simulink model "etb_Model"  (R2019b)
settings: Solver=FixedStepAuto  StartTime=0.0  StopTime=6  FixedStep=.001  RelTol=1e-3
undefined symbols (not defined in the file or in its folder): DiscIntNeverNeededParam
libraries: simulink x1
settings Model: Creator=Nick  LastModifiedBy=starw

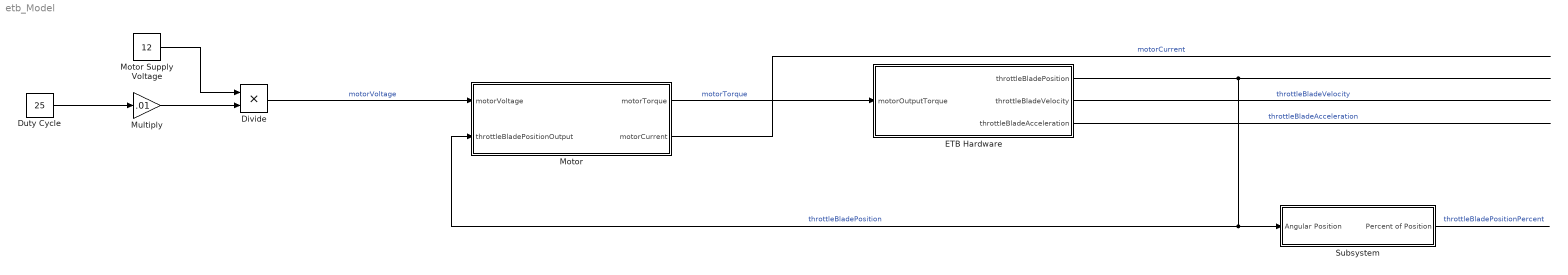
== system etb_Model ==
  Divide : Product  Inputs=**
  "Duty Cycle " : Constant  Value=25
  ETB Hardware : Subsystem
  Motor : Subsystem
  Motor Supply Voltage : Constant  Value=12
  Multiply : Gain  Gain=.01
  Subsystem : Subsystem
  wires:
  ETB Hardware/2(throttleBladeVelocity) -> ?  "throttleBladeVelocity"
  ETB Hardware/3(throttleBladeAcceleration) -> ?  "throttleBladeAcceleration"
  Motor/1(motorTorque) -> ETB Hardware/1(motorOutputTorque)  "motorTorque"
  Motor/2(motorCurrent) -> ?  "motorCurrent"
  ETB Hardware/1(throttleBladePosition) -> Subsystem/1(Angular Position), Motor/2(throttleBladePositionOutput)  "throttleBladePosition"
  Divide/1 -> Motor/1(motorVoltage)  "motorVoltage"
  Multiply/1 -> Divide/2
  Motor Supply Voltage/1 -> Divide/1
  "Duty Cycle "/1 -> Multiply/1
  Subsystem/1(Percent of Position) -> ?  "throttleBladePositionPercent"

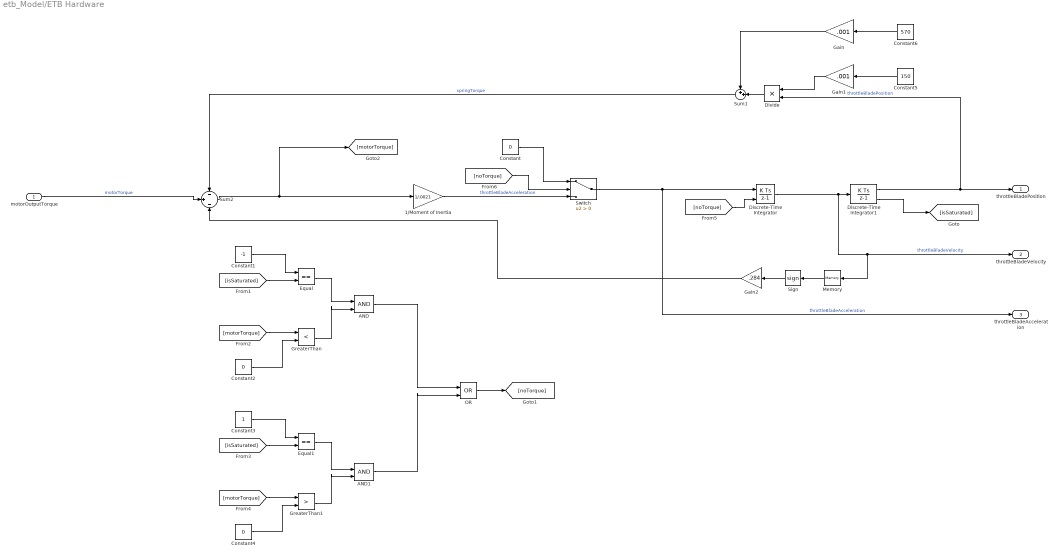
== system etb_Model/ETB Hardware ==
  motorOutputTorque : Inport
  1/Moment of Inertia : Gain  Gain=1/.0021
  AND : Logic  IconShape=distinctive  AllPortsSameDT=off  OutDataTypeStr=boolean
  AND1 : Logic  IconShape=distinctive  AllPortsSameDT=off  OutDataTypeStr=boolean
  Constant : Constant  Value=0
  Constant1 : Constant  Value=-1
  Constant2 : Constant  Value=0
  Constant3 : Constant
  Constant4 : Constant  Value=0
  Constant5 : Constant  Value=150
  Constant6 : Constant  Value=570
  Discrete-Time Integrator : DiscreteIntegrator  ExternalReset=level  SampleTime=-1  ICPrevOutput=DiscIntNeverNeededParam  ICPrevScaledInput=DiscIntNeverNeededParam
  Discrete-Time Integrator1 : DiscreteIntegrator  InitialCondition=0.109955  SampleTime=-1  LimitOutput=on  UpperSaturationLimit=1.5708  LowerSaturationLimit=0.109955  ShowSaturationPort=on  ICPrevOutput=DiscIntNeverNeededParam  ICPrevScaledInput=DiscIntNeverNeededParam
  Divide : Product  Inputs=**
  Equal : RelationalOperator  Operator===  OutDataTypeStr=boolean  RndMeth=Simplest
  Equal1 : RelationalOperator  Operator===  OutDataTypeStr=boolean  RndMeth=Simplest
  Gain : Gain  Gain=.001
  Gain1 : Gain  Gain=.001
  Gain2 : Gain  Gain=.284
  GreaterThan : RelationalOperator  Operator=<  OutDataTypeStr=boolean  RndMeth=Simplest
  GreaterThan1 : RelationalOperator  Operator=>  OutDataTypeStr=boolean  RndMeth=Simplest
  Memory : Memory
  OR : Logic  Operator=OR  IconShape=distinctive  AllPortsSameDT=off  OutDataTypeStr=boolean
  Sign : Signum
  Sum1 : Sum  Inputs=++|
  Sum2 : Sum  Inputs=-|+|-
  Switch : Switch  Criteria=u2 > Threshold
  throttleBladePosition : Outport
  throttleBladeVelocity : Outport  Port=2
  throttleBladeAcceleration : Outport  Port=3
  wires:
  Constant5/1 -> Gain1/1
  Gain1/1 -> Divide/1
  Constant6/1 -> Gain/1
  motorOutputTorque/1 -> Sum2/2  "motorTorque"
  Sum1/1 -> Sum2/1  "springTorque"
  Switch/1 -> Discrete-Time Integrator/1, throttleBladeAcceleration/1  "throttleBladeAcceleration"
  Discrete-Time Integrator/1 -> Memory/1, throttleBladeVelocity/1, Discrete-Time Integrator1/1  "throttleBladeVelocity"
  Discrete-Time Integrator1/1 -> throttleBladePosition/1, Divide/2  "throttleBladePosition"
  Divide/1 -> Sum1/2
  Gain/1 -> Sum1/1
  Sum2/1 -> 1/Moment of Inertia/1, [motorTorque]
  Constant1/1 -> Equal/1
  Equal/1 -> AND/1
  Discrete-Time Integrator1/2 -> [isSaturated]
  OR/1 -> [noTorque]
  [isSaturated] -> Equal/2
  GreaterThan/1 -> AND/2
  Constant2/1 -> GreaterThan/2
  [motorTorque] -> GreaterThan/1
  [motorTorque] -> GreaterThan1/1
  Constant4/1 -> GreaterThan1/2
  [isSaturated] -> Equal1/2
  Constant3/1 -> Equal1/1
  Equal1/1 -> AND1/1
  GreaterThan1/1 -> AND1/2
  AND/1 -> OR/1
  AND1/1 -> OR/2
  [noTorque] -> Discrete-Time Integrator/2
  1/Moment of Inertia/1 -> Switch/3  "throttleBladeAcceleration"
  [noTorque] -> Switch/2
  Constant/1 -> Switch/1
  Gain2/1 -> Sum2/3
  Memory/1 -> Sign/1
  Sign/1 -> Gain2/1

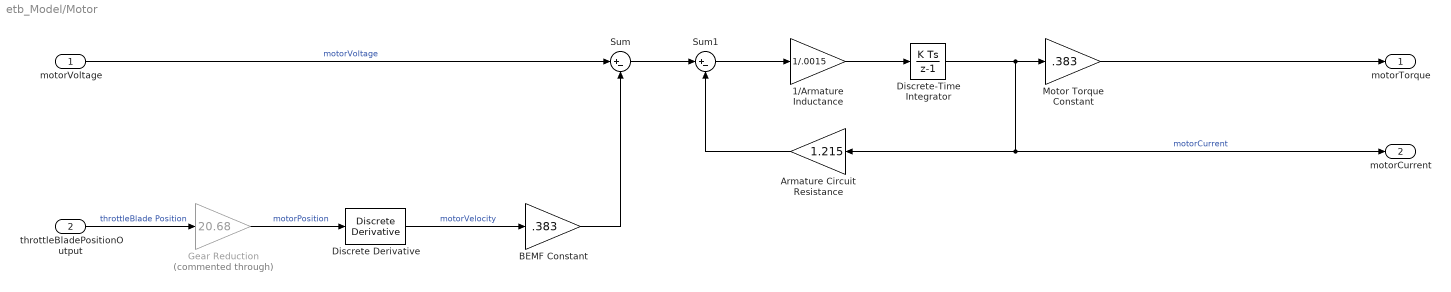
== system etb_Model/Motor ==
  motorVoltage : Inport
  throttleBladePositionOutput : Inport  Port=2
  1/Armature Inductance : Gain  Gain=1/.0015
  Armature Circuit Resistance : Gain  Gain=1.215
  BEMF Constant : Gain  Gain=.383
  Discrete Derivative : simulink/Discrete/Discrete Derivative  gainval=1.0  ICPrevScaledInput=0.0  OutMin=[]  OutMax=[]  OutDataType=fixdt(1, 16)  OutScaling=2^-10  DoSatur=off
  Discrete-Time Integrator : DiscreteIntegrator  SampleTime=-1  ICPrevOutput=DiscIntNeverNeededParam  ICPrevScaledInput=DiscIntNeverNeededParam
  Gear Reduction : Gain  Commented=through  Gain=20.68
  Motor Torque Constant : Gain  Gain=.383
  Sum : Sum  Inputs=|+-
  Sum1 : Sum  Inputs=|+-
  motorTorque : Outport
  motorCurrent : Outport  Port=2
  wires:
  Discrete-Time Integrator/1 -> Motor Torque Constant/1, motorCurrent/1, Armature Circuit Resistance/1  "motorCurrent"
  Motor Torque Constant/1 -> motorTorque/1
  motorVoltage/1 -> Sum/1  "motorVoltage"
  Armature Circuit Resistance/1 -> Sum1/2
  Sum1/1 -> 1/Armature Inductance/1
  1/Armature Inductance/1 -> Discrete-Time Integrator/1
  Sum/1 -> Sum1/1
  BEMF Constant/1 -> Sum/2
  throttleBladePositionOutput/1 -> Gear Reduction/1  "throttleBlade Position"
  Gear Reduction/1 -> Discrete Derivative/1  "motorPosition"
  Discrete Derivative/1 -> BEMF Constant/1  "motorVelocity"

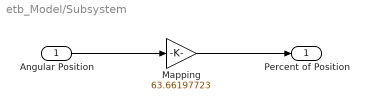
== system etb_Model/Subsystem ==
  Angular Position : Inport
  Mapping : Gain  Gain=63.66197723  OutMin=0  OutMax=100
  Percent of Position : Outport
  wires:
  Angular Position/1 -> Mapping/1
  Mapping/1 -> Percent of Position/1
